simulink library "ESTS_TFX"  (R2024b)
settings: Solver=VariableStepAuto  StartTime=0.0  StopTime=10.0  RelTol=1e-3
undefined symbols (not defined in the file or in its folder): ESTS_TFX_c_TiSample_s, ESTS_TFX_p_TauFiltDif_s, p_JyWhl_kgm2, p_RadWhlDynFr_m, p_RadWhlDynRe_m, p_RatGearFr_na, p_RatGearRe_na
libraries: VUT_lib x1
settings Model: Creator=blatak  LastModifiedBy=blatak
settings ModelReferenceCC: EnableRefExpFcnMdlSchedulingChecks=on
settings RTWCC: GPUComputeCapability=3.5

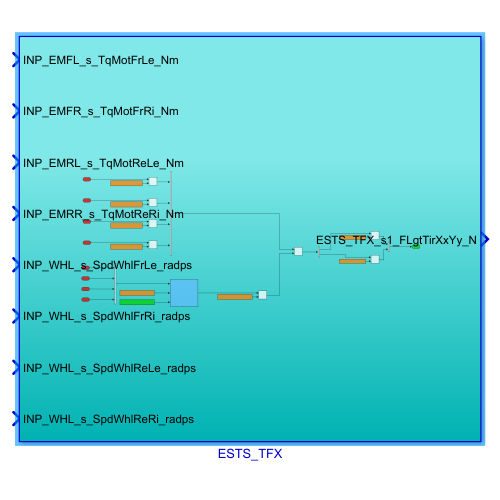
[thumbnail: Simulink's stored preview of the top-level diagram]
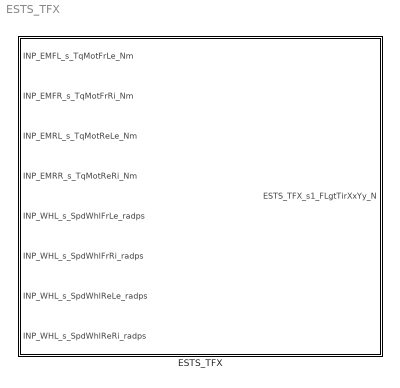
== system ESTS_TFX ==
  ESTS_TFX : Subsystem

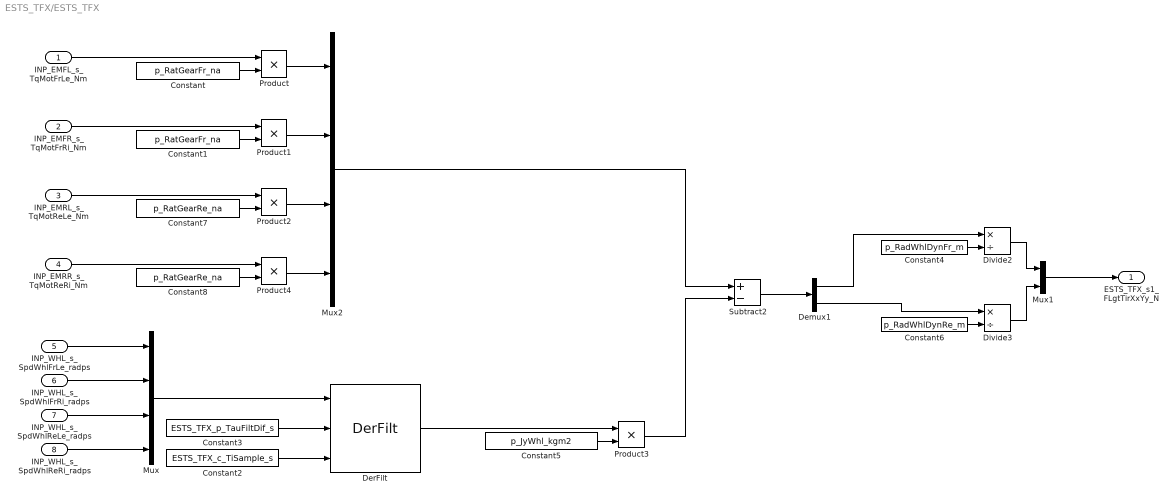
== system ESTS_TFX/ESTS_TFX ==
  INP_EMFL_s_TqMotFrLe_Nm : Inport  Description=INP Front electric motor torque - value after basic processing
  INP_EMFR_s_TqMotFrRi_Nm : Inport  Description=INP Rear electric motor torque - value after basic processing  Port=2
  INP_EMRL_s_TqMotReLe_Nm : Inport  Port=3
  INP_EMRR_s_TqMotReRi_Nm : Inport  Port=4
  INP_WHL_s_SpdWhlFrLe_radps : Inport  Description=INP wheel speed FL  Port=5
  INP_WHL_s_SpdWhlFrRi_radps : Inport  Description=INP wheel speed FR  Port=6
  INP_WHL_s_SpdWhlReLe_radps : Inport  Description=INP wheel speed RL  Port=7
  INP_WHL_s_SpdWhlReRi_radps : Inport  Description=INP wheel speed RR  Port=8
  Constant : Constant  Description=Overall gear ratio for front electric motor  Value=p_RatGearFr_na
  Constant1 : Constant  Description=Overall gear ratio for rear electric motor  Value=p_RatGearFr_na
  Constant2 : Constant  Description=Sample time for low pass filter  Value=ESTS_TFX_c_TiSample_s
  Constant3 : Constant  Value=ESTS_TFX_p_TauFiltDif_s
  Constant4 : Constant  Description=Parameter - front wheel dynamic radius  Value=p_RadWhlDynFr_m
  Constant5 : Constant  Description=Parameter - wheel moment of inertia  Value=p_JyWhl_kgm2
  Constant6 : Constant  Description=Parameter - rear wheel dynamic radius  Value=p_RadWhlDynRe_m
  Constant7 : Constant  Description=Overall gear ratio for front electric motor  Value=p_RatGearRe_na
  Constant8 : Constant  Description=Overall gear ratio for front electric motor  Value=p_RatGearRe_na
  Demux1 : Demux  Outputs=2
  DerFilt : VUT_lib/DerFilt  SystemSampleTime=-1  VariantActivationTime=update diagram  AllowFlexibleInterface=on  Latency=0  AutoFrameSizeCalculation=off
  Divide2 : Product  Inputs=*/
  Divide3 : Product  Inputs=*/
  Mux : Mux
  Mux1 : Mux  Inputs=2
  Mux2 : Mux
  Product{,1..4} (5 alike) : Product
  Subtract2 : Sum  Inputs=+-
  ESTS_TFX_s1_FLgtTirXxYy_N : Outport
  wires:
  INP_EMFL_s_TqMotFrLe_Nm/1 -> Product/1
  Constant/1 -> Product/2
  INP_EMFR_s_TqMotFrRi_Nm/1 -> Product1/1
  Constant1/1 -> Product1/2
  INP_WHL_s_SpdWhlFrLe_radps/1 -> Mux/1
  INP_WHL_s_SpdWhlFrRi_radps/1 -> Mux/2
  INP_WHL_s_SpdWhlReLe_radps/1 -> Mux/3
  INP_WHL_s_SpdWhlReRi_radps/1 -> Mux/4
  Product/1 -> Mux2/1
  Product1/1 -> Mux2/2
  Mux/1 -> DerFilt/1
  Constant2/1 -> DerFilt/3
  Constant3/1 -> DerFilt/2
  DerFilt/1 -> Product3/1
  Constant5/1 -> Product3/2
  Product3/1 -> Subtract2/2
  Subtract2/1 -> Demux1/1
  Demux1/1 -> Divide2/1
  Demux1/2 -> Divide3/1
  Constant4/1 -> Divide2/2
  Constant6/1 -> Divide3/2
  Divide2/1 -> Mux1/1
  Divide3/1 -> Mux1/2
  Mux1/1 -> ESTS_TFX_s1_FLgtTirXxYy_N/1
  INP_EMRL_s_TqMotReLe_Nm/1 -> Product2/1
  INP_EMRR_s_TqMotReRi_Nm/1 -> Product4/1
  Constant7/1 -> Product2/2
  Constant8/1 -> Product4/2
  Product2/1 -> Mux2/3
  Product4/1 -> Mux2/4
  Mux2/1 -> Subtract2/1
